simulink model "simple1"  (R2021b)
settings: Solver=VariableStepAuto  StartTime=0.0  StopTime=10.0  RelTol=1e-3
settings Model: Creator=fzy  LastModifiedBy=fzy

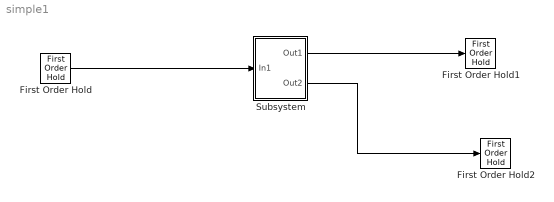
== system simple1 ==
  First Order Hold : FirstOrderHold  ErrorTolerance=inf
  First Order Hold1 : FirstOrderHold  ErrorTolerance=inf
  First Order Hold2 : FirstOrderHold  ErrorTolerance=inf
  Subsystem : Subsystem
  wires:
  First Order Hold/1 -> Subsystem/1(In1)
  Subsystem/1(Out1) -> First Order Hold1/1
  Subsystem/2(Out2) -> First Order Hold2/1

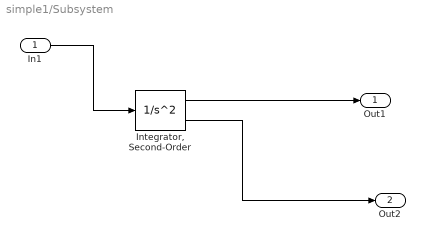
== system simple1/Subsystem ==
  In1 : Inport
  "Integrator, Second-Order" : SecondOrderIntegrator
  Out1 : Outport
  Out2 : Outport  Port=2
  wires:
  "Integrator, Second-Order"/2 -> Out2/1
  In1/1 -> "Integrator, Second-Order"/1
  "Integrator, Second-Order"/1 -> Out1/1
